simulink model "tutorial4"  (Simulink 2.20)
settings: Solver=ode5  StartTime=0.0  StopTime=tstop  FixedStep=tstep  MaxStep=tstep  RelTol=1e-3  AbsTol=1e-3
settings Model: SaveTime=off  SaveOutput=off  ConsistencyChecking=off  RTWPlaceOutputsASAP=off

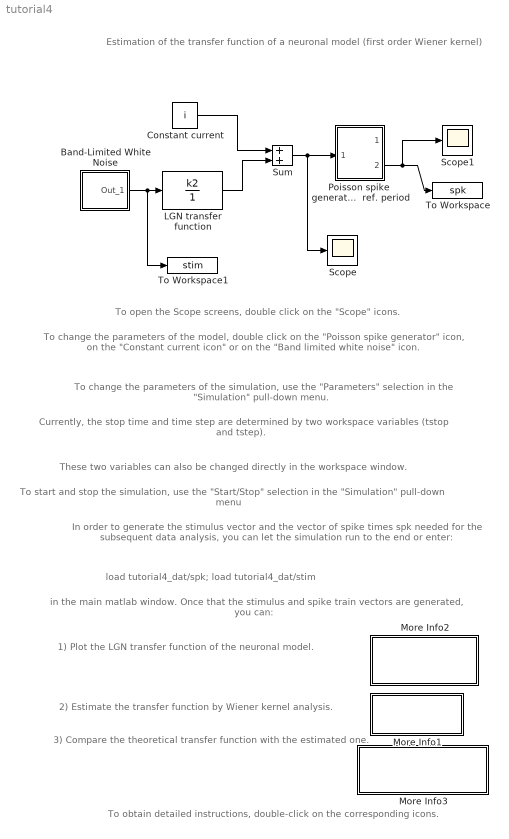
== system tutorial4 ==
  note: Estimation of the transfer function of a neuronal model
      | (first order Wiener kernel)
  note: To open the Scope screens, double click on the "Scope" icons.
  note: To change the parameters of the model, double click on the
      | "Poisson spike generator" icon, on the "Constant current icon"
      | or on the "Band limited white noise" icon.
  note: To change the parameters of the simulation, use the "Parameters"
      | selection in the "Simulation" pull-down menu.
  note: Currently, the stop time and time step are determined by two
      | workspace variables (tstop and tstep).
  note: These two variables can also be changed directly in the
      | workspace window.
  note: In order to generate the stimulus vector and the vector of spike times
      | spk needed for the subsequent data analysis, you can let the simulation
      | run to the end or enter:
  note: To start and stop the simulation, use the "Start/Stop"
      | selection in the "Simulation" pull-down menu
  note: To obtain detailed instructions, double-click on the corresponding
      | icons.
  note: 3) Compare the theoretical transfer function with
      | the estimated one.
  note: 2) Estimate  the transfer function by Wiener
      | kernel analysis.
  note: 1) Plot the LGN transfer function of the
      | neuronal model.
  note: in the main matlab window. Once that the stimulus and spike train
      | vectors are generated, you can:
  note: load tutorial4_dat/spk; load tutorial4_dat/stim
  Band-Limited White Noise : Subsystem  mask(Discrete time white noise. ){@1=tstep, @2=0.1, @3=[23341]}
      mask prompts: @1 "time step [msec]"; @2 "standard deviation [nA]"; @3 "random seed"
      mask help: Discrete time white noise
      mask init:
      | dt = @1; sigma = @2; seed = @3; r = rand(1,12); r2 = [r(1),r;r,r(12)]; t =[1:13;1:13];
      mask Help: Generates a sequence of normally distributed random numbers with standard deviation sigma
      mask Display: plot(t(:),r2(:))
  Constant current : Constant  Value=i  mask(constant current){@1=0.3}
      mask prompts: @1 "constant current value [nA]"
      mask help: Parameter
      mask init:
      | i = @1;
      mask Help: Provides a constant input current
  LGN transfer function : DiscreteFilter  Numerator=k2  Denominator=1  SampleTime=dt  mask(LGN transfer function){@1=5.5, @2=tstep, @3=1500}
      mask prompts: @1 "cut-off frequency [Hz]"; @2 "time step [msec]"; @3 "time constant [msec]"
      mask help: Parameters
      mask init:
      | omega_c = @1*2*pi; dt = @2; tau = @3*1e-3; b = sqrt(omega_c^2 + tau^(-2)) ; tv = [0:dt:512]; tv_s = tv*1e-3; k2 = tv_s.*(tau + 0.5*(1-tau*b)*tv_s).*exp(-b*tv_s); k2 = k2/norm(k2);
      mask Display: plot(tv,k2);
  More Info1 : Subsystem
      mask Display: disp('First order\nWiener kernel')
  More Info2 : Subsystem
      mask Display: disp('Transfer function\nof an LGN\nrelay cell')
  More Info3 : Subsystem
      mask Display: disp('Comparison between\ntrue and estimated\ntransfer function')
  Poisson spike  generator with  ref. period : Subsystem  mask(I&F p. thres., ref. per.){@1=tstep, @2=10, @3=.5, @4=1}
      mask prompts: @1 "time step [msec]"; @2 "mean threshold [mV]"; @3 "Capacitance [nF]"; @4 "refractory period [msec]"
      mask help: Parameters
      mask init:
      | dt = @1; thres = @2; C = @3; ref = @4;
      mask Help: For a detailled description of the model, please type 'help piandfr' in the main matlab window
      mask Display: disp('Vm \n\n spikes')
  Scope : Scope
      settings: TickLabels=on  TimeRange=500.000000  YMin=-0.600000  YMax=0.600000  SaveToWorkspace=off  SaveName=ScopeData
  Scope1 : Scope
      settings: TickLabels=on  TimeRange=500.000000  YMin=-2.000000  YMax=2.000000  SaveToWorkspace=off  SaveName=ScopeData
  Sum : Sum  Inputs=++
  To Workspace : ToWorkspace  VariableName=spk  SampleTime=0
      settings: Buffer=ceil(tstop/tstep)
  To Workspace1 : ToWorkspace  VariableName=stim  SampleTime=0
      settings: Buffer=ceil(tstop/tstep)
  wires:
  Band-Limited White Noise/1(Out_1) -> LGN transfer function/1, To Workspace1/1
  LGN transfer function/1 -> Sum/2
  Constant current/1 -> Sum/1
  Sum/1 -> Poisson spike  generator with  ref. period/1(in_1), Scope/1
  Poisson spike  generator with  ref. period/2(out_1) -> Scope1/1, To Workspace/1

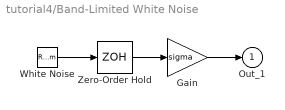
== system tutorial4/Band-Limited White Noise ==
  Gain : Gain  Gain=sigma
  White Noise : RandomNumber  Mean=0  Variance=1  Seed=seed  SampleTime=-1
  Zero-Order Hold : ZeroOrderHold  SampleTime=dt
  Out_1 : Outport  Port=1  InitialOutput=0
  wires:
  Zero-Order Hold/1 -> Gain/1
  Gain/1 -> Out_1/1
  White Noise/1 -> Zero-Order Hold/1

== system tutorial4/More Info1 ==
  note: To estimate the transfer function by Wiener kernel
      | analysis, enter:
  note: wiener1(stim,spk,tstep)
  note: in the workspace window.
  note: Note the high level of noise in the estimate of the impulse
      | response. This is caused by a too small sampling step.
  note: To obtain a better estimate by resampling at a lower frequency, enter:
  note: wiener1(stim,spk,tstep, 20,128,bartlett(128),64,'none')
  note: 20 = resampling step (only every 20th point is taken into account)
  note: 128 = number of frequency component computed (the resampling step
      | is 20*tstep = 10 ms, corresponding to 100 Hz sampling frequency
      | and thus the resolution is 100/128 Hz).
  note: The additional parameters are:
  note: bartlett(128) = window for the data
  note: 64 = overlap between adjacent data sets
  note: 'none' = detrending option in the Fast Fourier computation (see
      | the matlab signal toolbox for more details).

== system tutorial4/More Info2 ==
  note: To plot the transfer function of an LGN relay cell,enter
  note: lgnfilt(1500,5.5,tstep);
  note: in the workspace window.
  note: The parameters are:
  note: 5.5= cut-off frequency of the LGN transfer function
  note: tstep = time step for the simulation
  note: 1500 = time constant of decay for the stim. ensemble

== system tutorial4/More Info3 ==
  note: To compare the theoretical transfer function with
      | the one computed by Wiener kernel analysis, enter:
  note: [tf2,t2] = wiener1(stim,spk,tstep, 20,128,bartlett(128),64,'none')
  note: [tf1, t1] = lgnfilt(1500,5.5,tstep)
  note: plot(t1,conv_fac*tf1,'g',t2,tf2);
  note: in the workspace window.
  note: The units conversion factor is given by:
  note: conv_fac = 1e3/(C*V*tstep*1e-3)
  note: where,
  note: C = 0.5 nF
  note: Vthres = 10 mV
  note: tstep = 0.5 msec

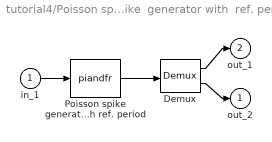
== system tutorial4/Poisson spike  generator with  ref. period ==
  in_1 : Inport  Port=1  PortWidth=-1  SampleTime=-1
  Demux : Demux  Outputs=2
  Poisson spike generator with ref. period : S-Function  FunctionName=piandfr  Parameters=dt,thres,C, ref  PortCounts=[]  SFunctionModules=''
  out_2 : Outport  Port=1  InitialOutput=0
  out_1 : Outport  Port=2  InitialOutput=0
  wires:
  Poisson spike generator with ref. period/1 -> Demux/1
  Demux/1 -> out_1/1
  Demux/2 -> out_2/1
  in_1/1 -> Poisson spike generator with ref. period/1
